simulink model "Examen1s"  (R2015b)
settings: Solver=VariableStepAuto  StartTime=0.0  StopTime=3  RelTol=1e-3
libraries: powerlib x10
settings Model: Creator=xmax1946  LastModifiedBy=xmax1946

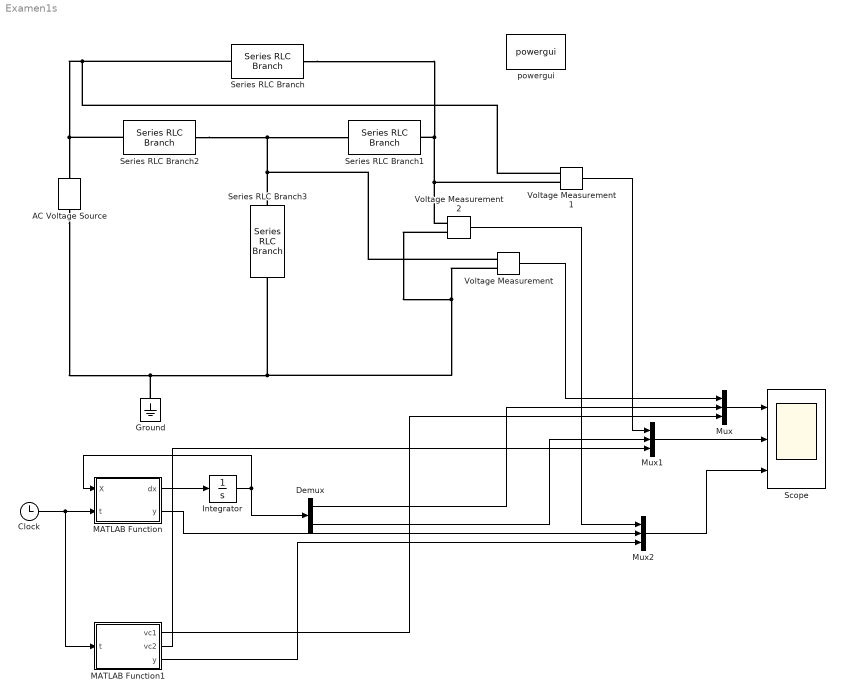
== system Examen1s ==
  AC Voltage Source : powerlib/Electrical Sources/AC Voltage Source  Amplitude=10  Phase=0  Frequency=1/(2*pi)  SampleTime=0  Measurements=None  BusType=swing  Pref=10e3  Qref=0  Qmin=-inf  Qmax=+inf
  Clock : Clock
  Demux : Demux  Outputs=2
  Ground : powerlib/Elements/Ground  LConnTagsString=a
  Integrator : Integrator  InitialCondition=[1;1]
  MATLAB Function : MATLAB Function  TreatAsAtomicUnit=on
  MATLAB Function1 : MATLAB Function  TreatAsAtomicUnit=on
  Mux : Mux  Inputs=3
  Mux1 : Mux  Inputs=3
  Mux2 : Mux  Inputs=3
  Scope : Scope  NumInputPorts=3
  Series RLC Branch : powerlib/Elements/Series RLC Branch  LConnTagsString=__new0  RConnTagsString=__new0  BranchType=C  Resistance=1  Inductance=1e-3  SetiL0=off  InitialCurrent=0  Capacitance=2  Setx0=on  InitialVoltage=1  Measurements=None
  Series RLC Branch1 : powerlib/Elements/Series RLC Branch  LConnTagsString=__new0  RConnTagsString=__new0  BranchType=R  Resistance=2  Inductance=1e-3  SetiL0=off  InitialCurrent=0  Capacitance=1e-6  Setx0=off  InitialVoltage=0  Measurements=None
  Series RLC Branch2 : powerlib/Elements/Series RLC Branch  LConnTagsString=__new0  RConnTagsString=__new0  BranchType=R  Resistance=1  Inductance=1e-3  SetiL0=off  InitialCurrent=0  Capacitance=1e-6  Setx0=off  InitialVoltage=0  Measurements=None
  Series RLC Branch3 : powerlib/Elements/Series RLC Branch  LConnTagsString=__new0  RConnTagsString=__new0  BranchType=C  Resistance=1  Inductance=1e-3  SetiL0=off  InitialCurrent=0  Capacitance=1  Setx0=on  InitialVoltage=1  Measurements=None
  Voltage Measurement : powerlib/Measurements/Voltage Measurement  PhasorSimulation=off  OutputType=Complex  PSBequivalent=0
  Voltage Measurement1 : powerlib/Measurements/Voltage Measurement  PhasorSimulation=off  OutputType=Complex  PSBequivalent=0
  Voltage Measurement2 : powerlib/Measurements/Voltage Measurement  PhasorSimulation=off  OutputType=Complex  PSBequivalent=0
  powergui : powerlib/powergui  Priority=1  SimulationMode=Discrete  SolverType=Tustin/Backward Euler (TBE)  SampleTime=50e-6  frequency=60  SPID=off  DisableSnubberDevices=off  DisableRonSwitches=off  DisableVfSwitches=off  SwTol=0  DisplayEquations=off  Interpol=off  ExternalGateDelay=off  methode=off  Ts=10  FunctionMessages=off  echomessages=off  HookPort=off  EnableUseOfTLC=off  x0status=blocks  frequencyindice=0.159154943091895  Pbase=100e6  ErrMax=1e-4  Iterations=50  UnitsV=kV  UnitsW=MW  buscounter=0  RestoreLinks=warning  ResistiveCurrentMeasurement=off  Frange=[0:2:500]  Ylog=off  Xlog=on  ShowGrid=off  save=off  variable=ZData  structure=0  ZoomFFT=off  StartTime=0.0  cycles=1  DisplayStyle=1  fundamental=60  FreqAxis=off  MaxFrequency=1000  frequencyindicesteady=1  RmsSteady=1  display=off
  wires:
  Clock/1 -> MATLAB Function1/1(t), MATLAB Function/2(t)
  MATLAB Function/1(dx) -> Integrator/1
  Integrator/1 -> Demux/1, MATLAB Function/1(X)
  Voltage Measurement/1 -> Mux/1
  Demux/1 -> Mux/2
  Voltage Measurement1/1 -> Mux1/1
  Mux/1 -> Scope/1
  Mux1/1 -> Scope/2
  Demux/2 -> Mux1/2
  Voltage Measurement2/1 -> Mux2/1
  Mux2/1 -> Scope/3
  MATLAB Function/2(y) -> Mux2/2
  MATLAB Function1/1(vc1) -> Mux/3
  MATLAB Function1/2(vc2) -> Mux1/3
  MATLAB Function1/3(y) -> Mux2/3
  connections:
  Series RLC Branch/LConn1 -- Voltage Measurement1/LConn1 -- Series RLC Branch2/LConn1 -- AC Voltage Source/RConn1
  Series RLC Branch/RConn1 -- Voltage Measurement2/LConn1 -- Voltage Measurement1/LConn2 -- Series RLC Branch1/RConn1
  Series RLC Branch2/RConn1 -- Voltage Measurement/LConn1 -- Series RLC Branch3/LConn1 -- Series RLC Branch1/LConn1
  AC Voltage Source/LConn1 -- Ground/LConn1 -- Voltage Measurement2/LConn2 -- Voltage Measurement/LConn2 -- Series RLC Branch3/RConn1

== matlab function Examen1s/MATLAB Function1 ==
  data: vc1 output; vc2 output; t input; y output
function [vc1,vc2,y] = fcn(t)

% vc1=(195*sin(t))/29 - (125*cos(t))/29 + (125*exp(-(7*t)/8)*cosh((33^(1/2)*t)/8))/29 + exp(-(7*t)/8)*(cosh((33^(1/2)*t)/8) - (5*33^(1/2)*sinh((33^(1/2)*t)/8))/33) - (267*33^(1/2)*exp(-(7*t)/8)*sinh((33^(1/2)*t)/8))/319;
% vc2=(35*sin(t))/29 - (15*cos(t))/29 + (15*exp(-(7*t)/8)*cosh((33^(1/2)*t)/8))/29 + exp(-(7*t)/8)*(cosh((33^(1/2)*t)/8) + (5*33^(1/2)*sinh((33^(1/2)*t)/8))/33) - (233*33^(1/2)*exp(-(7*t)/8)*sinh((33^(1/2)*t)/8))/957;
% y=(15*cos(t))/29 + (255*sin(t))/29 - (15*exp(-(7*t)/8)*cosh((33^(1/2)*t)/8))/29 - exp(-(7*t)/8)*(cosh((33^(1/2)*t)/8) + (5*33^(1/2)*sinh((33^(1/2)*t)/8))/33) + (233*33^(1/2)*exp(-(7*t)/8)*sinh((33^(1/2)*t)/8))/957;
vc1=0.10169962188284187823603029454696/(3060513257434037/1125899906842624)^(0.15692966918274642296182719292119*t)*(316912650057057350374175801344.0/(7804582818978274949762008801.0*log(3060513257434037/1125899906842624)^2 + 316912650057057350374175801344.0) - (562949953421312.0*exp(0.15692966918274642296182719292119*t*log(3060513257434037/1125899906842624))*(562949953421312.0*cos(t) - 88343549956849.0*log(3060513257434037/1125899906842624)*sin(t)))/(7804582818978274949762008801.0*log(3060513257434037/1125899906842624)^2 + 316912650057057350374175801344.0)) + 1.2833494518006402777357964290646/(3060513257434037/1125899906842624)^(1.5930703308172535770381728070788*t) - 0.28334945180064027773579642906464/(3060513257434037/1125899906842624)^(0.15692966918274642296182719292119*t) + 14.898300378117158235467740621324/(3060513257434037/1125899906842624)^(1.5930703308172535770381728070788*t)*(1/(2.5378730789301937519996681619218*log(3060513257434037/1125899906842624)^2 + 1.0) - (1.0*exp(1.5930703308172535770381728070788*t*log(3060513257434037/1125899906842624))*(cos(t) - 1.5930703308172535770381728070788*log(3060513257434037/1125899906842624)*sin(t)))/(2.5378730789301937519996681619218*log(3060513257434037/1125899906842624)^2 + 1.0)) - 0.00000000000000005685188545793526317011185647545/(3060513257434037/1125899906842624)^(0.15692966918274642296182719292119*t)*(1/(2.5378730789301937519996681619218*log(3060513257434037/1125899906842624)^2 + 1.0) - (1.0*exp(1.5930703308172535770381728070788*t*log(3060513257434037/1125899906842624))*(cos(t) - 1.5930703308172535770381728070788*log(3060513257434037/1125899906842624)*sin(t)))/(2.5378730789301937519996681619218*log(3060513257434037/1125899906842624)^2 + 1.0)) - 0.00000000000000005685188545793526317011185647545/(3060513257434037/1125899906842624)^(1.5930703308172535770381728070788*t)*(316912650057057350374175801344.0/(7804582818978274949762008801.0*log(3060513257434037/1125899906842624)^2 + 316912650057057350374175801344.0) - (562949953421312.0*exp(0.15692966918274642296182719292119*t*log(3060513257434037/1125899906842624))*(562949953421312.0*cos(t) - 88343549956849.0*log(3060513257434037/1125899906842624)*sin(t)))/(7804582818978274949762008801.0*log(3060513257434037/1125899906842624)^2 + 316912650057057350374175801344.0));
vc2=0.23888351606645324075473452364512/(3060513257434037/1125899906842624)^(1.5930703308172535770381728070788*t) - 0.27317948961235608612206770241426/(3060513257434037/1125899906842624)^(0.15692966918274642296182719292119*t)*(316912650057057350374175801344.0/(7804582818978274949762008801.0*log(3060513257434037/1125899906842624)^2 + 316912650057057350374175801344.0) - (562949953421312.0*exp(0.15692966918274642296182719292119*t*log(3060513257434037/1125899906842624))*(562949953421312.0*cos(t) - 88343549956849.0*log(3060513257434037/1125899906842624)*sin(t)))/(7804582818978274949762008801.0*log(3060513257434037/1125899906842624)^2 + 316912650057057350374175801344.0)) + 0.76111648393354675924526547635488/(3060513257434037/1125899906842624)^(0.15692966918274642296182719292119*t) + 2.7731794896123561050726961883927/(3060513257434037/1125899906842624)^(1.5930703308172535770381728070788*t)*(1/(2.5378730789301937519996681619218*log(3060513257434037/1125899906842624)^2 + 1.0) - (1.0*exp(1.5930703308172535770381728070788*t*log(3060513257434037/1125899906842624))*(cos(t) - 1.5930703308172535770381728070788*log(3060513257434037/1125899906842624)*sin(t)))/(2.5378730789301937519996681619218*log(3060513257434037/1125899906842624)^2 + 1.0)) - 0.0000000000000000094753142429892105283519760792417/(3060513257434037/1125899906842624)^(0.15692966918274642296182719292119*t)*(1/(2.5378730789301937519996681619218*log(3060513257434037/1125899906842624)^2 + 1.0) - (1.0*exp(1.5930703308172535770381728070788*t*log(3060513257434037/1125899906842624))*(cos(t) - 1.5930703308172535770381728070788*log(3060513257434037/1125899906842624)*sin(t)))/(2.5378730789301937519996681619218*log(3060513257434037/1125899906842624)^2 + 1.0)) - 0.0000000000000000094753142429892105283519760792417/(3060513257434037/1125899906842624)^(1.5930703308172535770381728070788*t)*(316912650057057350374175801344.0/(7804582818978274949762008801.0*log(3060513257434037/1125899906842624)^2 + 316912650057057350374175801344.0) - (562949953421312.0*exp(0.15692966918274642296182719292119*t*log(3060513257434037/1125899906842624))*(562949953421312.0*cos(t) - 88343549956849.0*log(3060513257434037/1125899906842624)*sin(t)))/(7804582818978274949762008801.0*log(3060513257434037/1125899906842624)^2 + 316912650057057350374175801344.0));
y= 10*sin(t) + 0.27317948961235608612206770241426/(3060513257434037/1125899906842624)^(0.15692966918274642296182719292119*t)*(316912650057057350374175801344.0/(7804582818978274949762008801.0*log(3060513257434037/1125899906842624)^2 + 316912650057057350374175801344.0) - (562949953421312.0*exp(0.15692966918274642296182719292119*t*log(3060513257434037/1125899906842624))*(562949953421312.0*cos(t) - 88343549956849.0*log(3060513257434037/1125899906842624)*sin(t)))/(7804582818978274949762008801.0*log(3060513257434037/1125899906842624)^2 + 316912650057057350374175801344.0)) - 0.23888351606645324075473452364512/(3060513257434037/1125899906842624)^(1.5930703308172535770381728070788*t) - 0.76111648393354675924526547635488/(3060513257434037/1125899906842624)^(0.15692966918274642296182719292119*t) - 2.7731794896123561050726961883927/(3060513257434037/1125899906842624)^(1.5930703308172535770381728070788*t)*(1/(2.5378730789301937519996681619218*log(3060513257434037/1125899906842624)^2 + 1.0) - (1.0*exp(1.5930703308172535770381728070788*t*log(3060513257434037/1125899906842624))*(cos(t) - 1.5930703308172535770381728070788*log(3060513257434037/1125899906842624)*sin(t)))/(2.5378730789301937519996681619218*log(3060513257434037/1125899906842624)^2 + 1.0)) + 0.0000000000000000094753142429892105283519760792417/(3060513257434037/1125899906842624)^(0.15692966918274642296182719292119*t)*(1/(2.5378730789301937519996681619218*log(3060513257434037/1125899906842624)^2 + 1.0) - (1.0*exp(1.5930703308172535770381728070788*t*log(3060513257434037/1125899906842624))*(cos(t) - 1.5930703308172535770381728070788*log(3060513257434037/1125899906842624)*sin(t)))/(2.5378730789301937519996681619218*log(3060513257434037/1125899906842624)^2 + 1.0)) + 0.0000000000000000094753142429892105283519760792417/(3060513257434037/1125899906842624)^(1.5930703308172535770381728070788*t)*(316912650057057350374175801344.0/(7804582818978274949762008801.0*log(3060513257434037/1125899906842624)^2 + 316912650057057350374175801344.0) - (562949953421312.0*exp(0.15692966918274642296182719292119*t*log(3060513257434037/1125899906842624))*(562949953421312.0*cos(t) - 88343549956849.0*log(3060513257434037/1125899906842624)*sin(t)))/(7804582818978274949762008801.0*log(3060513257434037/1125899906842624)^2 + 316912650057057350374175801344.0));

== matlab function Examen1s/MATLAB Function ==
  data: dx output; X input; y output; t input
function [dx,y] = fss(X,t)
c1=1;
c2=2;
r1=1;
r2=2;

A=[(-1/c1)*((r1+r2)/(r1*r2)),-1/(c1*r2)
    -1/(c2*r2),-1/(c2*r2)];
B=[(1/c1)*((r2+r1)/(r1*r2));1/(c2*r2)];
C=[0 -1];
D=1;

u=10*sin(t);
dx=A*X+B*u;
y=C*X+D*u;
